simulink model "noiseModel"  (R2023b)
settings: Solver=FixedStepAuto  StartTime=0.0  StopTime=60  FixedStep=1e-4  RelTol=1e-12  AbsTol=1e-12
libraries: dspsrcs4 x1, dspsigops x1
settings Model: SimulationMode=accelerator  Creator=anigo  LastModifiedBy=anigo
settings DataIOCC: SaveFormat=Array  SignalLogging=off  DSMLogging=off  ReturnWorkspaceOutputs=off

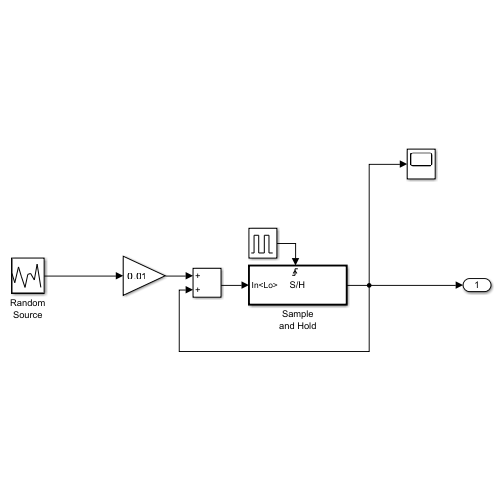
[thumbnail: Simulink's stored preview of the top-level diagram]
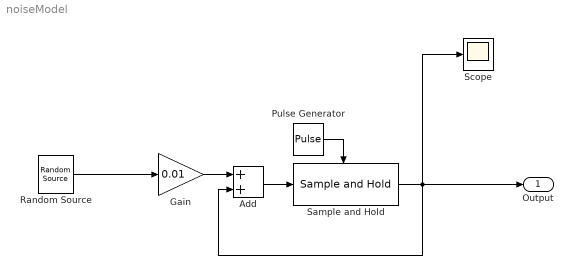
== system noiseModel ==
  Add : Sum
  Gain : Gain  Gain=0.01
  Pulse Generator : DiscretePulseGenerator  PulseType=Time based  Period=0.01  PulseWidth=5
  Random Source : dspsrcs4/Random Source  SrcType=Gaussian  NormMethod=Ziggurat  CltLength=12  MinVal=0  MaxVal=1  MeanVal=0  VarVal=1  RepMode=Not repeatable  rawSeed=1  IsInherit=off  SampMode=Discrete  SampTime=0.01  SampFrame=1  DataType=Double  OutComplex=Real  OutputFrames=off
  Sample and Hold : dspsigops/Sample and Hold  trig=Rising edge  initCond=0  latchinput=on
  Scope : Scope
  Output : Outport
  wires:
  Pulse Generator/1 -> Sample and Hold/Trigger
  Gain/1 -> Add/1
  Add/1 -> Sample and Hold/1
  Sample and Hold/1 -> Scope/1, Output/1, Add/2
  Random Source/1 -> Gain/1
